simulink model "controllermodel"  (R2020b)
settings: Solver=FixedStepDiscrete  StartTime=0.0  StopTime=10.0  FixedStep=1/100  RelTol=1e-3
undefined symbols (not defined in the file or in its folder): DiscIntNeverNeededParam
libraries: simulink_extras x4, pid_lib x1
settings Model: Creator=janik  LastModifiedBy=Ralf Senger
settings OptimizationCC: DefaultParameterBehavior=Inlined  EnhancedBackFolding=on  PassReuseOutputArgsAs=Individual arguments  ZeroExternalMemoryAtStartup=off  ZeroInternalMemoryAtStartup=off  OptimizeBlockOrder=speed  DifferentSizesBufferReuse=on  OptimizationCustomize=off  EfficientTunableParamExpr=on
settings DebuggingCC: ParameterTunabilityLossMsg=error
settings SFSimCC: MATLABDynamicMemAlloc=off  SimTargetLang=C++
settings RTWCC: Description=Embedded Coder  SystemTargetFile=ert.tlc  GenCodeOnly=on  TemplateMakefile=ert_default_tmf  GenerateReport=on  Toolchain=GNU Tools for ARM Embedded Processors  LaunchReport=on  TargetLang=C++
settings CodeAppCC: ForceParamTrailComments=on  IgnoreCustomStorageClasses=off  OperatorAnnotations=on  SimulinkDataObjDesc=on  SFDataObjDesc=on  MATLABFcnDesc=on  InsertBlockDesc=on
settings ERTTargetCC: TargetLangStandard=C++03 (ISO)  GenerateSampleERTMain=on  CodeInterfacePackaging=C++ class  SupportVariableSizeSignals=on  InlinedParameterPlacement=NonHierarchical  RootIOFormat=Structure reference  ERTCustomFileTemplate=example_file_process.tlc

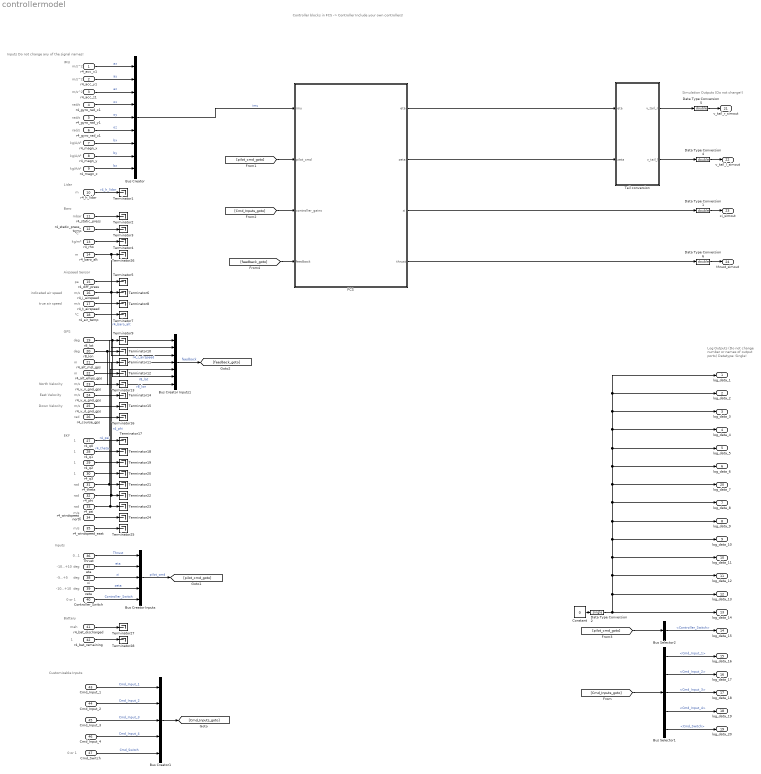
== system controllermodel ==
  note: EKF
  note: Lidar
  note: m/s
  note: Baro
  note: rad
  note: rad
  note: indicated air speed
  note: Inputs
      | Do not change any of the
      | signal names!
  note: m/s
  note: 1
  note: Controller blocks in FCS -> Controller
      |
      | Include your own controllers!
  note: -10...+10
  note: Log Outputs
      | (Do not change
      | number or names
      | of output ports)
      | Datatype: Single!
  note: deg
  note: pa
  note: East Velocity
  note: m
  note: kg/A/s²
  note: m
  note: m/s^2
  note: m/s^2
  note: true air speed
  note: Airpseed Sensor
  note: 1
  note: Inputs
  note: m/s
  note: mbar
  note: m
  note: deg
  note: kg/A/s²
  note: deg
  note: Battery
  note: rad/s
  note: 0 or 1
  note: 1
  note: rad/s
  note: mah
  note: Customizable Inputs
  note: m/s
  note: m/s
  note: m/s
  note: m/s^2
  note: North Velocity
  note: °C
  note: rad/s
  note: °C
  note: rad
  note: -5...+5
  note: m
  note: kg/A/s²
  note: 1
  note: 0...1
  note: deg
  note: rad
  note: Down Velocity
  note: IMU
  note: -10...+10
  note: deg
  note: 1
  note: Simulation Outputs
      | (Do not change!)
  note: 0 or 1
  note: GPS
  note: m/s
  note: kg/m³
  r4_acc_x1 : Inport  OutDataTypeStr=single  Unit=m/s^2  PortDimensions=1  SampleTime=1/50  Interpolate=off
  r4_acc_y1 : Inport  Port=2  OutDataTypeStr=single  Unit=m/s^2  PortDimensions=1  SampleTime=1/50  Interpolate=off
  r4_acc_z1 : Inport  Port=3  OutDataTypeStr=single  Unit=m/s^2  PortDimensions=1  SampleTime=1/50  Interpolate=off
  r4_gyro_rad_x1 : Inport  Port=4  OutDataTypeStr=single  Unit=rad/s  PortDimensions=1  SampleTime=1/50  Interpolate=off
  r4_gyro_rad_y1 : Inport  Port=5  OutDataTypeStr=single  Unit=rad/s  PortDimensions=1  SampleTime=1/50  Interpolate=off
  r4_gyro_rad_z1 : Inport  Port=6  OutDataTypeStr=single  Unit=rad/s  PortDimensions=1  SampleTime=1/50  Interpolate=off  LockScale=on
  r4_magn_x : Inport  Port=7  OutDataTypeStr=single  Unit=kg/A/s^2  PortDimensions=1  SampleTime=1/50  Interpolate=off
  r4_magn_y : Inport  Port=8  OutDataTypeStr=single  Unit=kg/A/s^2  PortDimensions=1  SampleTime=1/50  Interpolate=off
  r4_magn_z : Inport  Port=9  OutDataTypeStr=single  Unit=kg/A/s^2  PortDimensions=1  SampleTime=1/50  Interpolate=off
  r4_h_lidar : Inport  Port=10  OutDataTypeStr=single  Unit=m  PortDimensions=1  SampleTime=1/50  Interpolate=off
  r4_static_press : Inport  Port=11  OutDataTypeStr=single  Unit=mbar  PortDimensions=1  SampleTime=1/50  Interpolate=off
  r4_static_press_temp : Inport  Port=12  OutDataTypeStr=single  Unit=°C  PortDimensions=1  SampleTime=1/50  Interpolate=off
  r4_rho : Inport  Port=13  OutDataTypeStr=single  Unit=kg/m^3  PortDimensions=1  SampleTime=1/50  Interpolate=off
  r4_baro_alt : Inport  Port=14  OutDataTypeStr=single  Unit=m  PortDimensions=1  SampleTime=1/50  Interpolate=off
  r4_diff_press : Inport  Port=15  OutDataTypeStr=single  Unit=Pa  PortDimensions=1  SampleTime=1/50  Interpolate=off
  r4_i_airspeed : Inport  Port=16  OutDataTypeStr=single  Unit=m/s  PortDimensions=1  SampleTime=1/50  Interpolate=off
  r4_t_airspeed : Inport  Port=17  OutDataTypeStr=single  Unit=m/s  PortDimensions=1  SampleTime=1/50  Interpolate=off
  r4_air_temp : Inport  Port=18  OutDataTypeStr=single  Unit=°C  PortDimensions=1  SampleTime=1/50  Interpolate=off
  r8_lat : Inport  Port=19  OutDataTypeStr=double  Unit=deg  PortDimensions=1  SampleTime=1/50  Interpolate=off
  r8_lon : Inport  Port=20  OutDataTypeStr=double  Unit=deg  PortDimensions=1  SampleTime=1/50  Interpolate=off
  r4_alt_msl_gps : Inport  Port=21  OutDataTypeStr=single  Unit=m  PortDimensions=1  SampleTime=1/50  Interpolate=off
  r4_alt_ellips_gps : Inport  Port=22  OutDataTypeStr=single  Unit=m  PortDimensions=1  SampleTime=1/50  Interpolate=off
  r4_v_n_gnd_gps : Inport  Port=23  OutDataTypeStr=single  Unit=m/s  PortDimensions=1  SampleTime=1/50  Interpolate=off
  r4_v_e_gnd_gps : Inport  Port=24  OutDataTypeStr=single  Unit=m/s  PortDimensions=1  SampleTime=1/50  Interpolate=off
  r4_v_d_gnd_gps : Inport  Port=25  OutDataTypeStr=single  Unit=m/s  PortDimensions=1  SampleTime=1/50  Interpolate=off
  r4_course_gps : Inport  Port=26  OutDataTypeStr=single  Unit=rad  PortDimensions=1  SampleTime=1/50  Interpolate=off
  r4_q0 : Inport  Port=27  OutMin=[-1]  OutMax=[1]  OutDataTypeStr=single  Unit=1  PortDimensions=1  SampleTime=1/50  Interpolate=off
  r4_q1 : Inport  Port=28  OutMin=[-1]  OutMax=[1]  OutDataTypeStr=single  Unit=1  PortDimensions=1  SampleTime=1/50  Interpolate=off
  r4_q2 : Inport  Port=29  OutMin=[-1]  OutMax=[1]  OutDataTypeStr=single  Unit=1  PortDimensions=1  SampleTime=1/50  Interpolate=off
  r4_q3 : Inport  Port=30  OutMin=[-1]  OutMax=[1]  OutDataTypeStr=single  Unit=one  PortDimensions=1  SampleTime=1/50  Interpolate=off
  r4_theta : Inport  Port=31  OutDataTypeStr=single  Unit=rad  PortDimensions=1  SampleTime=1/50  Interpolate=off
  r4_phi : Inport  Port=32  OutDataTypeStr=single  Unit=rad  PortDimensions=1  SampleTime=1/50  Interpolate=off
  r4_psi : Inport  Port=33  OutDataTypeStr=single  Unit=rad  PortDimensions=1  SampleTime=1/50  Interpolate=off
  r4_windspeed_north : Inport  Port=34  OutDataTypeStr=single  Unit=m/s  PortDimensions=1  SampleTime=1/50  Interpolate=off
  r4_windspeed_east : Inport  Port=35  OutDataTypeStr=single  Unit=m/s  PortDimensions=1  SampleTime=1/50  Interpolate=off
  Thrust : Inport  Port=36  OutDataTypeStr=single  PortDimensions=1  SampleTime=1/50  Interpolate=off
  eta : Inport  Port=37  OutDataTypeStr=single  Unit=deg  PortDimensions=1  SampleTime=1/50  Interpolate=off
  xi : Inport  Port=38  OutDataTypeStr=single  Unit=deg  PortDimensions=1  SampleTime=1/50  Interpolate=off
  zeta : Inport  Port=39  OutDataTypeStr=single  Unit=deg  PortDimensions=1  SampleTime=1/50  Interpolate=off
  Controller_Switch : Inport  Port=40  OutDataTypeStr=single  PortDimensions=1  SampleTime=1/50  Interpolate=off
  r4_bat_discharged : Inport  Port=41  OutDataTypeStr=single  Unit=mA*hr  PortDimensions=1  SampleTime=1/50  Interpolate=off
  r4_bat_remaining : Inport  Port=42  OutDataTypeStr=single  PortDimensions=1  SampleTime=1/50  Interpolate=off
  Cmd_Input_1 : Inport  Port=43  OutDataTypeStr=single  PortDimensions=1  SampleTime=1/50  Interpolate=off
  Cmd_Input_2 : Inport  Port=44  OutDataTypeStr=single  PortDimensions=1  SampleTime=1/50  Interpolate=off
  Cmd_Input_3 : Inport  Port=45  OutDataTypeStr=single  PortDimensions=1  SampleTime=1/50  Interpolate=off
  Cmd_Input_4 : Inport  Port=46  OutDataTypeStr=single  PortDimensions=1  SampleTime=1/50  Interpolate=off
  Cmd_Switch : Inport  Port=47  OutDataTypeStr=single  PortDimensions=1  SampleTime=1/50  Interpolate=off
  Bus Creator : BusCreator  Inputs=9
  Bus Creator Inputs : BusCreator  Inputs=5
  Bus Creator Inputs1 : BusCreator  Inputs=7
  Bus Creator1 : BusCreator  Inputs=5
  Bus Selector1 : BusSelector  OutputSignals=Cmd_Input_1,Cmd_Input_2,Cmd_Input_3,Cmd_Input_4,Cmd_Switch
  Bus Selector2 : BusSelector  OutputSignals=Controller_Switch
  Constant : Constant  Value=0
  Data Type Conversion{1,4..6} (4 alike) : DataTypeConversion  OutDataTypeStr=double  RndMeth=Nearest
  Data Type Conversion2 : DataTypeConversion  OutDataTypeStr=single  RndMeth=Nearest
  FCS : Subsystem
  Tail conversion : Subsystem
  Terminator{1..28} (28 alike) : Terminator
  log_data_1 : Outport  OutDataTypeStr=single  VectorParamsAs1DForOutWhenUnconnected=off
  log_data_2 : Outport  Port=2  OutDataTypeStr=single  VectorParamsAs1DForOutWhenUnconnected=off
  log_data_3 : Outport  Port=3  OutDataTypeStr=single  VectorParamsAs1DForOutWhenUnconnected=off
  log_data_4 : Outport  Port=4  OutDataTypeStr=single  VectorParamsAs1DForOutWhenUnconnected=off
  log_data_5 : Outport  Port=5  OutDataTypeStr=single  VectorParamsAs1DForOutWhenUnconnected=off
  log_data_6 : Outport  Port=6  OutDataTypeStr=single  VectorParamsAs1DForOutWhenUnconnected=off
  log_data_8 : Outport  Port=7  OutDataTypeStr=single  VectorParamsAs1DForOutWhenUnconnected=off
  log_data_9 : Outport  Port=8  OutDataTypeStr=single  VectorParamsAs1DForOutWhenUnconnected=off
  log_data_10 : Outport  Port=9  OutDataTypeStr=single  VectorParamsAs1DForOutWhenUnconnected=off
  log_data_11 : Outport  Port=10  OutDataTypeStr=single  VectorParamsAs1DForOutWhenUnconnected=off
  log_data_12 : Outport  Port=11  OutDataTypeStr=single  VectorParamsAs1DForOutWhenUnconnected=off
  log_data_13 : Outport  Port=12  OutDataTypeStr=single  VectorParamsAs1DForOutWhenUnconnected=off
  log_data_14 : Outport  Port=13  OutDataTypeStr=single  VectorParamsAs1DForOutWhenUnconnected=off
  log_data_15 : Outport  Port=14  OutDataTypeStr=single  VectorParamsAs1DForOutWhenUnconnected=off
  log_data_16 : Outport  Port=15  OutDataTypeStr=single  VectorParamsAs1DForOutWhenUnconnected=off
  log_data_17 : Outport  Port=16  OutDataTypeStr=single  VectorParamsAs1DForOutWhenUnconnected=off
  log_data_18 : Outport  Port=17  OutDataTypeStr=single  VectorParamsAs1DForOutWhenUnconnected=off
  log_data_19 : Outport  Port=18  OutDataTypeStr=single  VectorParamsAs1DForOutWhenUnconnected=off
  log_data_20 : Outport  Port=19  OutDataTypeStr=single  VectorParamsAs1DForOutWhenUnconnected=off
  log_data_7 : Outport  Port=20  OutDataTypeStr=single  VectorParamsAs1DForOutWhenUnconnected=off
  v_tail_r_simout : Outport  Port=21  OutDataTypeStr=double  Unit=rad  VectorParamsAs1DForOutWhenUnconnected=off
  v_tail_l_simout : Outport  Port=22  OutDataTypeStr=double  Unit=rad  VectorParamsAs1DForOutWhenUnconnected=off
  xi_simout : Outport  Port=23  OutDataTypeStr=double  Unit=rad  VectorParamsAs1DForOutWhenUnconnected=off
  thrust_simout : Outport  Port=24  OutDataTypeStr=double  VectorParamsAs1DForOutWhenUnconnected=off
  wires:
  r4_bat_discharged/1 -> Terminator27/1
  [feedback_goto] -> FCS/4(feedback)
  Cmd_Switch/1 -> Bus Creator1/5  "Cmd_Switch"
  r4_theta/1 -> Bus Creator Inputs1/1, Terminator21/1  "r4_theta"
  Bus Selector1/5 -> log_data_20/1  "<Cmd_Switch>"
  r4_baro_alt/1 -> Bus Creator Inputs1/2, Terminator26/1  "r4_baro_alt"
  Data Type Conversion1/1 -> xi_simout/1
  r4_v_n_gnd_gps/1 -> Terminator13/1
  r4_static_press/1 -> Terminator2/1
  r4_h_lidar/1 -> Terminator1/1  "r4_h_lidar"
  Tail conversion/2(v_tail_l) -> Data Type Conversion4/1
  r4_q0/1 -> Terminator17/1
  FCS/4(thrust) -> Data Type Conversion6/1
  r4_alt_ellips_gps/1 -> Terminator12/1
  [Cmd_Inputs_goto] -> FCS/3(controller_gains)
  r4_gyro_rad_x1/1 -> Bus Creator/4  "ox"
  Data Type Conversion2/1 -> log_data_9/1, log_data_8/1, log_data_7/1, log_data_4/1, log_data_3/1, log_data_1/1, log_data_2/1, log_data_5/1, log_data_6/1, log_data_10/1, log_data_11/1, log_data_12/1, log_data_13/1, log_data_14/1
  r4_phi/1 -> Terminator22/1, Bus Creator Inputs1/4  "r4_phi"
  r4_i_airspeed/1 -> Bus Creator Inputs1/3, Terminator6/1  "r4_i_airspeed"
  FCS/2(zeta) -> Tail conversion/2(zeta)
  Bus Creator Inputs1/1 -> [feedback_goto]  "feedback"
  r4_psi/1 -> Terminator23/1, Bus Creator Inputs1/5  "r4_psi"
  r4_magn_x/1 -> Bus Creator/7  "bx"
  Data Type Conversion5/1 -> v_tail_r_simout/1
  r4_course_gps/1 -> Terminator16/1
  r4_magn_y/1 -> Bus Creator/8  "by"
  [pilot_cmd_goto] -> Bus Selector2/1
  r4_v_e_gnd_gps/1 -> Terminator14/1
  Bus Selector1/1 -> log_data_16/1  "<Cmd_Input_1>"
  Tail conversion/1(v_tail_r) -> Data Type Conversion5/1
  r4_t_airspeed/1 -> Terminator8/1
  r4_acc_y1/1 -> Bus Creator/2  "ay"
  Cmd_Input_1/1 -> Bus Creator1/1  "Cmd_Input_1"
  FCS/1(eta) -> Tail conversion/1(eta)
  Bus Selector1/4 -> log_data_19/1  "<Cmd_Input_4>"
  xi/1 -> Bus Creator Inputs/3  "xi"
  r4_windspeed_north/1 -> Terminator24/1
  r4_gyro_rad_z1/1 -> Bus Creator/6  "oz"
  eta/1 -> Bus Creator Inputs/2  "eta"
  Bus Selector2/1 -> log_data_15/1  "<Controller_Switch>"
  zeta/1 -> Bus Creator Inputs/4  "zeta"
  Bus Creator Inputs/1 -> [pilot_cmd_goto]  "pilot_cmd"
  Cmd_Input_2/1 -> Bus Creator1/2  "Cmd_Input_2"
  Data Type Conversion4/1 -> v_tail_l_simout/1
  r8_lat/1 -> Terminator9/1, Bus Creator Inputs1/6  "r8_lat"
  Cmd_Input_3/1 -> Bus Creator1/3  "Cmd_Input_3"
  r4_q1/1 -> Terminator18/1
  r4_q3/1 -> Terminator20/1
  r4_rho/1 -> Terminator4/1
  Data Type Conversion6/1 -> thrust_simout/1
  Controller_Switch/1 -> Bus Creator Inputs/5  "Controller_Switch"
  [pilot_cmd_goto] -> FCS/2(pilot_cmd)
  Thrust/1 -> Bus Creator Inputs/1  "Thrust"
  Cmd_Input_4/1 -> Bus Creator1/4  "Cmd_Input_4"
  FCS/3(xi) -> Data Type Conversion1/1
  r4_air_temp/1 -> Terminator7/1
  r4_acc_z1/1 -> Bus Creator/3  "az"
  r4_acc_x1/1 -> Bus Creator/1  "ax"
  r4_static_press_temp/1 -> Terminator3/1
  r8_lon/1 -> Terminator10/1, Bus Creator Inputs1/7  "r8_lon"
  Constant/1 -> Data Type Conversion2/1
  Bus Creator/1 -> FCS/1(imu)  "imu"
  r4_windspeed_east/1 -> Terminator25/1
  r4_bat_remaining/1 -> Terminator28/1
  Bus Selector1/2 -> log_data_17/1  "<Cmd_Input_2>"
  r4_magn_z/1 -> Bus Creator/9  "bz"
  r4_q2/1 -> Terminator19/1
  [Cmd_Inputs_goto] -> Bus Selector1/1
  r4_gyro_rad_y1/1 -> Bus Creator/5  "oy"
  r4_diff_press/1 -> Terminator5/1
  Bus Selector1/3 -> log_data_18/1  "<Cmd_Input_3>"
  r4_alt_msl_gps/1 -> Terminator11/1
  r4_v_d_gnd_gps/1 -> Terminator15/1
  Bus Creator1/1 -> [Cmd_Inputs_goto]

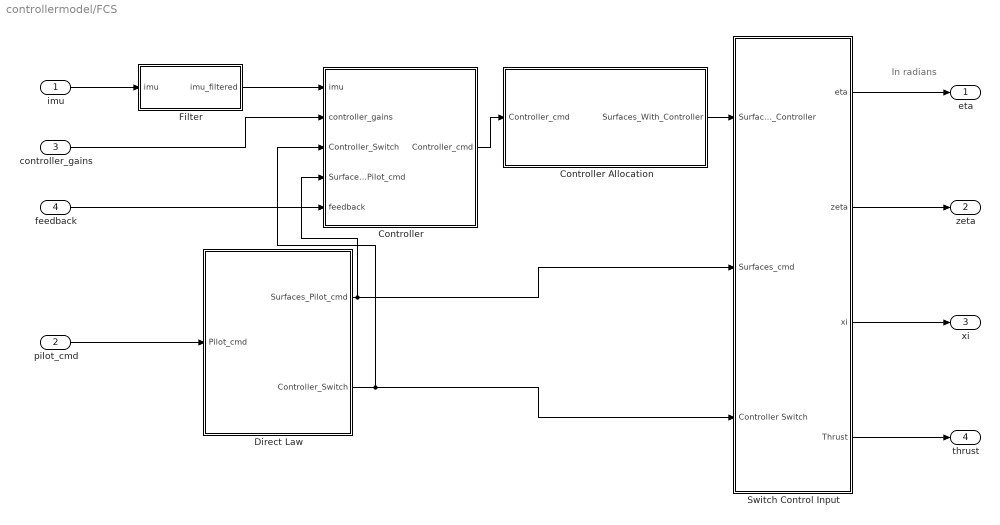
== system controllermodel/FCS ==
  note: In radians
  imu : Inport
  pilot_cmd : Inport  Port=2
  controller_gains : Inport  Port=3
  feedback : Inport  Port=4
  Controller : Subsystem
  Controller Allocation : Subsystem
  Direct Law : Subsystem
  Filter : Subsystem
  Switch Control Input : Subsystem
  eta : Outport  Unit=rad
  zeta : Outport  Port=2  Unit=rad
  xi : Outport  Port=3  Unit=rad
  thrust : Outport  Port=4  Unit=rad
  wires:
  Controller Allocation/1(Surfaces_With_Controller) -> Switch Control Input/1(Surfaces_With_Controller)
  pilot_cmd/1 -> Direct Law/1(Pilot_cmd)
  imu/1 -> Filter/1(imu)
  Switch Control Input/4(Thrust) -> thrust/1
  Switch Control Input/2(zeta) -> zeta/1
  Switch Control Input/1(eta) -> eta/1
  Switch Control Input/3(xi) -> xi/1
  Filter/1(imu_filtered) -> Controller/1(imu)
  Direct Law/2(Controller_Switch) -> Switch Control Input/3(Controller Switch), Controller/3(Controller_Switch)
  controller_gains/1 -> Controller/2(controller_gains)
  Direct Law/1(Surfaces_Pilot_cmd) -> Switch Control Input/2(Surfaces_cmd), Controller/4(Surfaces_Pilot_cmd)
  Controller/1(Controller_cmd) -> Controller Allocation/1(Controller_cmd)
  feedback/1 -> Controller/5(feedback)

== system controllermodel/Tail conversion ==
  eta : Inport  Unit=rad
  zeta : Inport  Port=2  Unit=rad
  Add1 : Sum  OutDataTypeStr=double
  Add2 : Sum  Inputs=+-  InputSameDT=on  OutDataTypeStr=double
  v_tail_r : Outport  Unit=rad
  v_tail_l : Outport  Port=2  Unit=rad
  wires:
  Add1/1 -> v_tail_l/1
  Add2/1 -> v_tail_r/1
  zeta/1 -> Add2/2, Add1/2
  eta/1 -> Add2/1, Add1/1

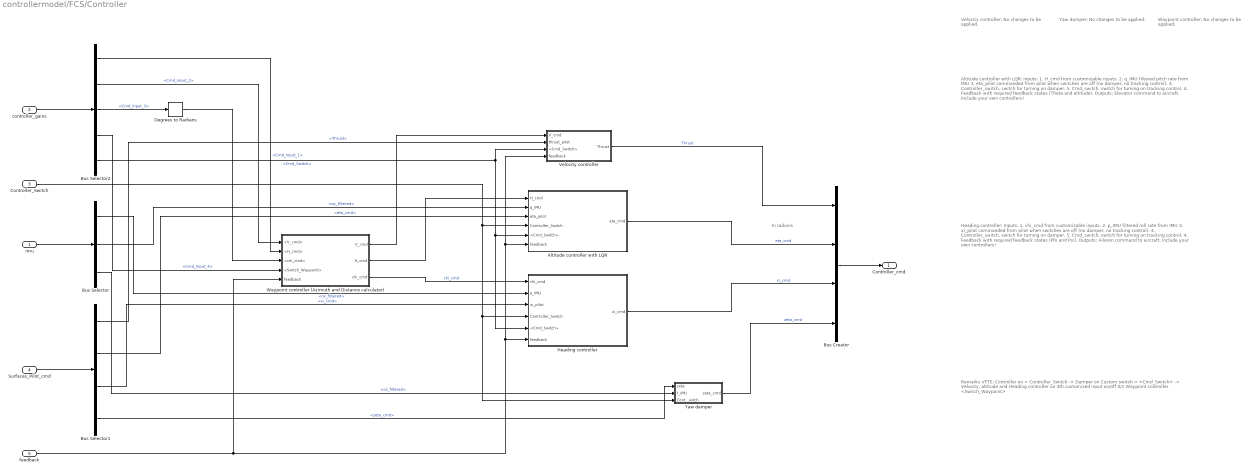
== system controllermodel/FCS/Controller ==
  note: Remarks VFTE:
      |
      | Controller on = Controller_Switch -> Damper on
      | Custom switch = <Cmd_Switch> -> Velocity, altitude and Heading controller on
      | 4th customized input on/off 0/1 Waypoint controller <Switch_Waypoint>
  note: In radians
  note: Veloctiy controller:
      |
      | No changes to be applied.
  note: Altitude controller with LQR:
      |
      | Inputs:
      |
      | 1. H_cmd from customizable inputs.
      | 2. q_IMU filtered pitch rate from IMU
      | 3. eta_pilot commanded from pilot when switches are off (no damper, no tracking control).
      | 4. Controller_switch, switch for turning on damper.
      | 5. Cmd_switch, switch for turning on tracking control.
      | 4. Feedback with required feedback states (Theta and altitude).
      |
      | Outputs:
      |
      | Elevator command to aircraft.
      |
      | Include your own controllers!
  note: Heading controller:
      |
      | Inputs:
      |
      | 1. chi_cmd from customizable inputs.
      | 2. p_IMU filtered roll rate from IMU
      | 3. xi_pilot commanded from pilot when switches are off (no damper, no tracking control).
      | 4. Controller_switch, switch for turning on damper.
      | 5. Cmd_switch, switch for turning on tracking control.
      | 4. Feedback with required feedback states (Phi and Psi).
      |
      | Outputs:
      |
      | Aileron command to aircraft.
      |
      | Include your own controllers!
  note: Yaw damper:
      |
      | No changes to be applied.
  note: Waypoint controller:
      |
      | No changes to be applied.
  imu : Inport
  controller_gains : Inport  Port=2
  Controller_Switch : Inport  Port=3
  Surfaces_Pilot_cmd : Inport  Port=4
  feedback : Inport  Port=5
  Altitude controller with LQR : Subsystem
  Bus Creator : BusCreator  Inputs=4
  Bus Selector : BusSelector  OutputSignals=ox_filtered,oy_filtered,oz_filtered
  Bus Selector1 : BusSelector  OutputSignals=Thrust,eta_cmd,xi_cmd,zeta_cmd
  Bus Selector2 : BusSelector  OutputSignals=Cmd_Input_1,Cmd_Input_2,Cmd_Input_3,Cmd_Input_4,Cmd_Switch
  Degrees to Radians : simulink_extras/Transformations/Degrees to Radians
  Heading controller : Subsystem
  Velocity controller : Subsystem
  Waypoint controller (Azimuth and Distance calculator) : Subsystem
  Yaw damper : Subsystem
  Controller_cmd : Outport
  wires:
  Bus Creator/1 -> Controller_cmd/1
  controller_gains/1 -> Bus Selector2/1
  Altitude controller with LQR/1(eta_cmd) -> Bus Creator/2  "eta_cmd"
  Bus Selector/3 -> Yaw damper/2(r_IMU)  "<oz_filtered>"
  Bus Selector/1 -> Heading controller/2(p_IMU)  "<ox_filtered>"
  Bus Selector/2 -> Altitude controller with LQR/2(q_IMU)  "<oy_filtered>"
  imu/1 -> Bus Selector/1
  Controller_Switch/1 -> Altitude controller with LQR/4(Controller_Switch), Yaw damper/3(Controller_Switch), Heading controller/4(Controller_Switch)
  Surfaces_Pilot_cmd/1 -> Bus Selector1/1
  Bus Selector1/2 -> Altitude controller with LQR/3(eta_pilot)  "<eta_cmd>"
  Bus Selector1/1 -> Velocity controller/2(thrust_pilot)  "<Thrust>"
  Bus Selector1/3 -> Heading controller/3(xi_pilot)  "<xi_cmd>"
  Bus Selector1/4 -> Yaw damper/1(zeta)  "<zeta_cmd>"
  feedback/1 -> Waypoint controller (Azimuth and Distance calculator)/5(feedback), Velocity controller/4(feedback), Altitude controller with LQR/6(feedback), Heading controller/6(feedback)
  Bus Selector2/1 -> Waypoint controller (Azimuth and Distance calculator)/2(<H_cmd>)  "<Cmd_Input_1>"
  Bus Selector2/2 -> Waypoint controller (Azimuth and Distance calculator)/1(<V_cmd>)  "<Cmd_Input_2>"
  Bus Selector2/3 -> Degrees to Radians/1  "<Cmd_Input_3>"
  Bus Selector2/4 -> Waypoint controller (Azimuth and Distance calculator)/4(<Switch_Waypoint>)  "<Cmd_Input_4>"
  Bus Selector2/5 -> Heading controller/5(<Cmd_Switch>), Altitude controller with LQR/5(<Cmd_Switch>), Velocity controller/3(<Cmd_Switch>)  "<Cmd_Switch>"
  Velocity controller/1(Thrust) -> Bus Creator/1  "Thrust"
  Heading controller/1(xi_cmd) -> Bus Creator/3  "xi_cmd"
  Yaw damper/1(zeta_cmd) -> Bus Creator/4  "zeta_cmd"
  Degrees to Radians/1 -> Waypoint controller (Azimuth and Distance calculator)/3(<chi_cmd>)
  Waypoint controller (Azimuth and Distance calculator)/3(chi_cmd) -> Heading controller/1(chi_cmd)  "chi_cmd"
  Waypoint controller (Azimuth and Distance calculator)/1(V_cmd) -> Velocity controller/1(V_cmd)
  Waypoint controller (Azimuth and Distance calculator)/2(H_cmd) -> Altitude controller with LQR/1(H_cmd)

== system controllermodel/FCS/Controller Allocation ==
  note: Do not change signal names
      | or saturation
  Controller_cmd : Inport
  Bus Creator : BusCreator  Inputs=4
  Bus Selector1 : BusSelector  OutputSignals=Thrust,eta_cmd,xi_cmd,zeta_cmd
  Saturation : Saturate  UpperLimit=deg2rad(10)  LowerLimit=deg2rad(-20)
  Saturation1 : Saturate  UpperLimit=deg2rad(5)  LowerLimit=deg2rad(-5)
  Saturation2 : Saturate  UpperLimit=deg2rad(10)  LowerLimit=deg2rad(-10)
  Saturation3 : Saturate  UpperLimit=1  LowerLimit=0
  Surfaces_With_Controller : Outport
  wires:
  Bus Creator/1 -> Surfaces_With_Controller/1
  Controller_cmd/1 -> Bus Selector1/1
  Bus Selector1/4 -> Saturation2/1  "<zeta_cmd>"
  Bus Selector1/3 -> Saturation1/1  "<xi_cmd>"
  Bus Selector1/2 -> Saturation/1  "<eta_cmd>"
  Bus Selector1/1 -> Saturation3/1  "<Thrust>"
  Saturation/1 -> Bus Creator/2  "eta_cmd"
  Saturation1/1 -> Bus Creator/3  "xi_cmd"
  Saturation2/1 -> Bus Creator/4  "zeta_cmd"
  Saturation3/1 -> Bus Creator/1  "Thrust"

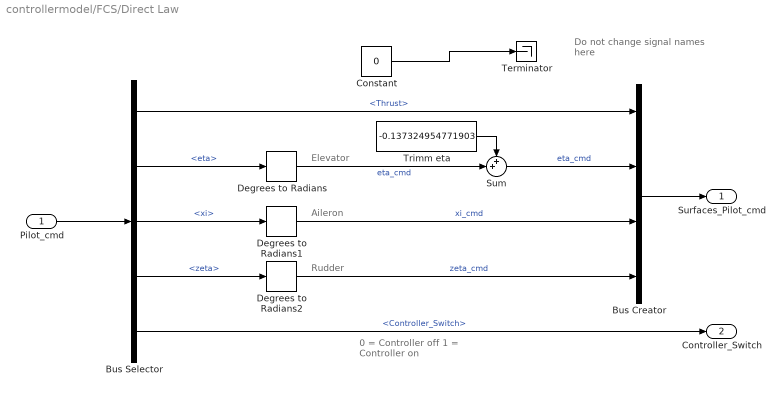
== system controllermodel/FCS/Direct Law ==
  note: Elevator
  note: 0 = Controller off
      | 1 = Controller on
  note: Do not change
      | signal names
      | here
  note: Aileron
  note: Rudder
  Pilot_cmd : Inport
  Bus Creator : BusCreator  Inputs=4
  Bus Selector : BusSelector  OutputSignals=Thrust,eta,xi,zeta,Controller_Switch
  Constant : Constant  Value=0
  Degrees to Radians : simulink_extras/Transformations/Degrees to Radians
  Degrees to Radians1 : simulink_extras/Transformations/Degrees to Radians
  Degrees to Radians2 : simulink_extras/Transformations/Degrees to Radians
  Sum : Sum  Inputs=++|
  Terminator : Terminator
  Trimm eta : Constant  Description=trim thrust  Value=-0.137324954771903  OutDataTypeStr=double
  Surfaces_Pilot_cmd : Outport
  Controller_Switch : Outport  Port=2
  wires:
  Pilot_cmd/1 -> Bus Selector/1
  Bus Selector/1 -> Bus Creator/1  "<Thrust>"
  Bus Selector/2 -> Degrees to Radians/1  "<eta>"
  Bus Selector/4 -> Degrees to Radians2/1  "<zeta>"
  Bus Selector/3 -> Degrees to Radians1/1  "<xi>"
  Bus Selector/5 -> Controller_Switch/1  "<Controller_Switch>"
  Bus Creator/1 -> Surfaces_Pilot_cmd/1
  Sum/1 -> Bus Creator/2  "eta_cmd"
  Degrees to Radians1/1 -> Bus Creator/3  "xi_cmd"
  Degrees to Radians2/1 -> Bus Creator/4  "zeta_cmd"
  Degrees to Radians/1 -> Sum/2  "eta_cmd"
  Trimm eta/1 -> Sum/1
  Constant/1 -> Terminator/1

== system controllermodel/FCS/Filter ==
  imu : Inport
  Bus Creator : BusCreator  Inputs=3
  Bus Selector : BusSelector  OutputSignals=ox,oy,oz
  ox_Filter : Subsystem
  oy_Filter : Subsystem
  oz_Filter : Subsystem
  imu_filtered : Outport
  wires:
  imu/1 -> Bus Selector/1
  Bus Selector/1 -> ox_Filter/1(<ox>)  "<ox>"
  ox_Filter/1(ox_filtered) -> Bus Creator/1  "ox_filtered"
  Bus Selector/2 -> oy_Filter/1(<oy>)  "<oy>"
  oy_Filter/1(oy_filtered) -> Bus Creator/2  "oy_filtered"
  Bus Selector/3 -> oz_Filter/1(<oz>)  "<oz>"
  oz_Filter/1(oz_filtered) -> Bus Creator/3  "oz_filtered"
  Bus Creator/1 -> imu_filtered/1

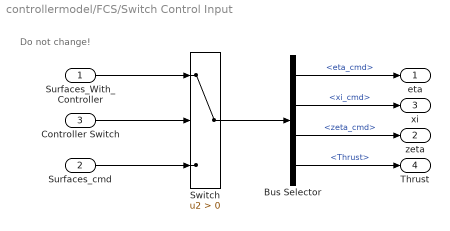
== system controllermodel/FCS/Switch Control Input ==
  note: Do not change!
  Surfaces_With_Controller : Inport
  Surfaces_cmd : Inport  Port=2
  Controller Switch : Inport  Port=3
  Bus Selector : BusSelector  OutputSignals=eta_cmd,xi_cmd,zeta_cmd,Thrust
  Switch : Switch  Criteria=u2 > Threshold
  eta : Outport
  zeta : Outport  Port=2
  xi : Outport  Port=3
  Thrust : Outport  Port=4
  wires:
  Surfaces_With_Controller/1 -> Switch/1
  Controller Switch/1 -> Switch/2
  Surfaces_cmd/1 -> Switch/3
  Switch/1 -> Bus Selector/1
  Bus Selector/1 -> eta/1  "<eta_cmd>"
  Bus Selector/2 -> xi/1  "<xi_cmd>"
  Bus Selector/3 -> zeta/1  "<zeta_cmd>"
  Bus Selector/4 -> Thrust/1  "<Thrust>"

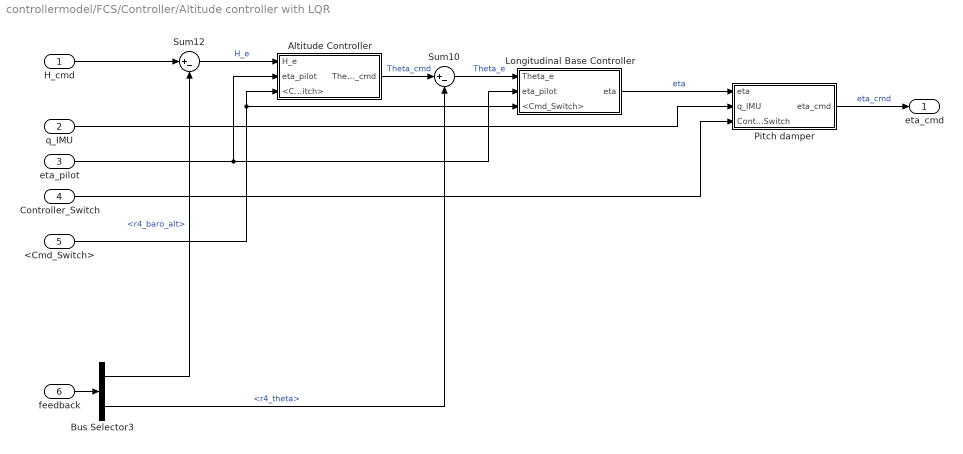
== system controllermodel/FCS/Controller/Altitude controller with LQR ==
  H_cmd : Inport
  q_IMU : Inport  Port=2
  eta_pilot : Inport  Port=3
  Controller_Switch : Inport  Port=4
  <Cmd_Switch> : Inport  Port=5
  feedback : Inport  Port=6
  Altitude Controller : Subsystem
  Bus Selector3 : BusSelector  OutputSignals=r4_baro_alt,r4_theta
  Longitudinal Base Controller : Subsystem
  Pitch damper : Subsystem
  Sum10 : Sum  Inputs=|+-
  Sum12 : Sum  Inputs=|+-
  eta_cmd : Outport
  wires:
  H_cmd/1 -> Sum12/1
  Pitch damper/1(eta_cmd) -> eta_cmd/1  "eta_cmd"
  Longitudinal Base Controller/1(eta) -> Pitch damper/1(eta)  "eta"
  Altitude Controller/1(Theta_cmd) -> Sum10/1  "Theta_cmd"
  Sum10/1 -> Longitudinal Base Controller/1(Theta_e)  "Theta_e"
  Sum12/1 -> Altitude Controller/1(H_e)  "H_e"
  q_IMU/1 -> Pitch damper/2(q_IMU)
  eta_pilot/1 -> Altitude Controller/2(eta_pilot), Longitudinal Base Controller/2(eta_pilot)
  Controller_Switch/1 -> Pitch damper/3(Controller_Switch)
  <Cmd_Switch>/1 -> Longitudinal Base Controller/3(<Cmd_Switch>), Altitude Controller/3(<Cmd_Switch>)
  feedback/1 -> Bus Selector3/1
  Bus Selector3/2 -> Sum10/2  "<r4_theta>"
  Bus Selector3/1 -> Sum12/2  "<r4_baro_alt>"

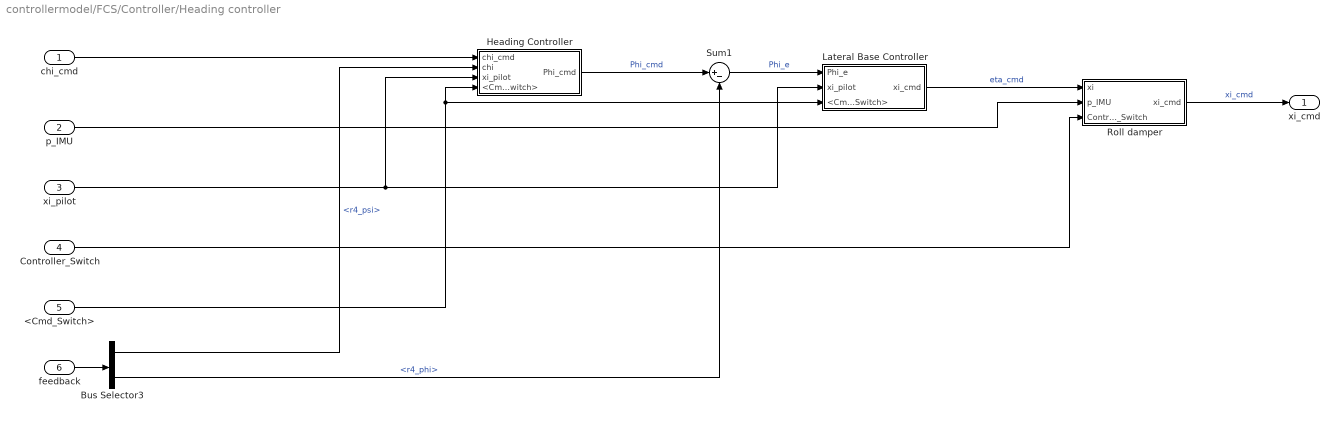
== system controllermodel/FCS/Controller/Heading controller ==
  chi_cmd : Inport
  p_IMU : Inport  Port=2
  xi_pilot : Inport  Port=3
  Controller_Switch : Inport  Port=4
  <Cmd_Switch> : Inport  Port=5
  feedback : Inport  Port=6
  Bus Selector3 : BusSelector  OutputSignals=r4_psi,r4_phi
  Heading Controller : Subsystem
  Lateral Base Controller : Subsystem
  Roll damper : Subsystem
  Sum1 : Sum  Inputs=|+-
  xi_cmd : Outport
  wires:
  Heading Controller/1(Phi_cmd) -> Sum1/1  "Phi_cmd"
  Roll damper/1(xi_cmd) -> xi_cmd/1  "xi_cmd"
  Lateral Base Controller/1(xi_cmd) -> Roll damper/1(xi)  "eta_cmd"
  Sum1/1 -> Lateral Base Controller/1(Phi_e)  "Phi_e"
  chi_cmd/1 -> Heading Controller/1(chi_cmd)
  p_IMU/1 -> Roll damper/2(p_IMU)
  xi_pilot/1 -> Heading Controller/3(xi_pilot), Lateral Base Controller/2(xi_pilot)
  Controller_Switch/1 -> Roll damper/3(Controller_Switch)
  <Cmd_Switch>/1 -> Heading Controller/4(<Cmd_Switch>), Lateral Base Controller/3(<Cmd_Switch>)
  Bus Selector3/2 -> Sum1/2  "<r4_phi>"
  feedback/1 -> Bus Selector3/1
  Bus Selector3/1 -> Heading Controller/2(chi)  "<r4_psi>"

== system controllermodel/FCS/Controller/Velocity controller ==
  V_cmd : Inport
  thrust_pilot : Inport  Port=2
  <Cmd_Switch> : Inport  Port=3
  feedback : Inport  Port=4
  Bus Selector3 : BusSelector  OutputSignals=r4_i_airspeed
  Sum14 : Sum  Inputs=|+-
  Velocity controller : Subsystem
  Thrust : Outport
  wires:
  Sum14/1 -> Velocity controller/1(V_e)  "V_e"
  Velocity controller/1(Thrust) -> Thrust/1  "Thrust"
  V_cmd/1 -> Sum14/1
  thrust_pilot/1 -> Velocity controller/2(thrust_pilot)
  <Cmd_Switch>/1 -> Velocity controller/3(<Cmd_Switch>)
  Bus Selector3/1 -> Sum14/2  "<r4_i_airspeed>"
  feedback/1 -> Bus Selector3/1

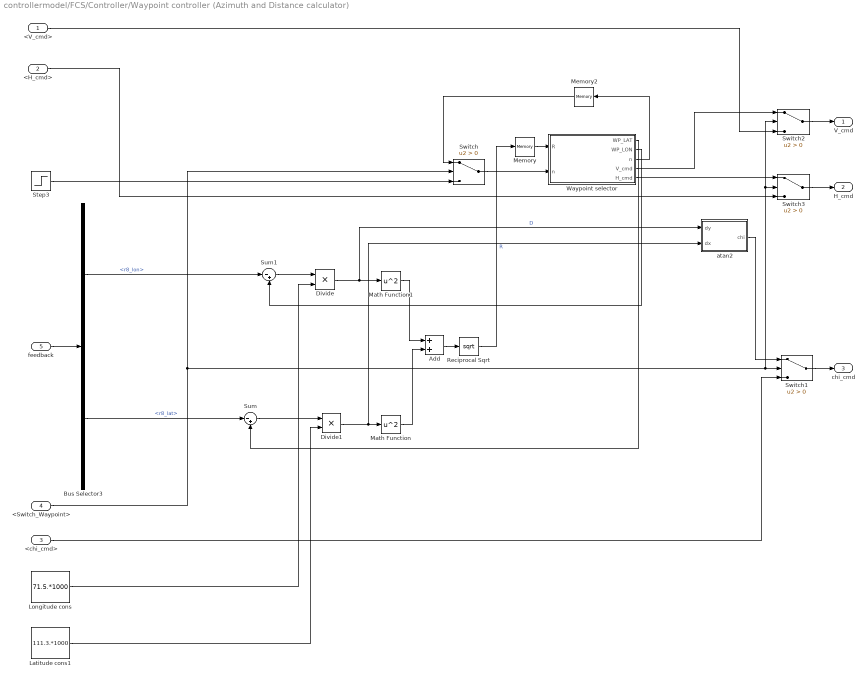
== system controllermodel/FCS/Controller/Waypoint controller (Azimuth and Distance calculator) ==
  <V_cmd> : Inport
  <H_cmd> : Inport  Port=2
  <chi_cmd> : Inport  Port=3
  <Switch_Waypoint> : Inport  Port=4
  feedback : Inport  Port=5
  Add : Sum
  Bus Selector3 : BusSelector  OutputSignals=r8_lon,r8_lat
  Divide : Product
  Divide1 : Product
  Latitude cons1 : Constant  Value=111.3.*1000
  Longitude cons : Constant  Value=71.5.*1000
  Math Function : Math  Operator=square  SaturateOnIntegerOverflow=on
  Math Function1 : Math  Operator=square  SaturateOnIntegerOverflow=on
  Memory : Memory
  Memory2 : Memory
  Reciprocal Sqrt : Sqrt  SaturateOnIntegerOverflow=on
  Step3 : Step  Time=0  Before=1  SampleTime=0.01
  Sum : Sum  Inputs=|-+
  Sum1 : Sum  Inputs=|-+
  Switch{,1..3} (4 alike) : Switch  Criteria=u2 > Threshold
  Waypoint selector : MATLAB Function  TreatAsAtomicUnit=on
  atan2 : MATLAB Function  TreatAsAtomicUnit=on
  V_cmd : Outport
  H_cmd : Outport  Port=2
  chi_cmd : Outport  Port=3
  wires:
  Longitude cons/1 -> Divide/2
  Sum1/1 -> Divide/1
  Sum/1 -> Divide1/1
  Latitude cons1/1 -> Divide1/2
  Divide1/1 -> atan2/2(dx), Math Function/1
  Divide/1 -> atan2/1(dy), Math Function1/1  "D"
  Math Function/1 -> Add/2
  Math Function1/1 -> Add/1
  Add/1 -> Reciprocal Sqrt/1
  Reciprocal Sqrt/1 -> Memory/1  "R"
  Waypoint selector/2(WP_LON) -> Sum1/2
  Switch/1 -> Waypoint selector/2("n ")
  Memory/1 -> Waypoint selector/1(R)
  Waypoint selector/1(WP_LAT) -> Sum/2
  Waypoint selector/3(n) -> Memory2/1
  Memory2/1 -> Switch/1
  Step3/1 -> Switch/3
  atan2/1(chi) -> Switch1/1
  Switch1/1 -> chi_cmd/1
  <Switch_Waypoint>/1 -> Switch2/2, Switch3/2, Switch1/2, Switch/2
  <chi_cmd>/1 -> Switch1/3
  Bus Selector3/1 -> Sum1/1  "<r8_lon>"
  Bus Selector3/2 -> Sum/1  "<r8_lat>"
  feedback/1 -> Bus Selector3/1
  Switch2/1 -> V_cmd/1
  Switch3/1 -> H_cmd/1
  <V_cmd>/1 -> Switch2/3
  <H_cmd>/1 -> Switch3/3
  Waypoint selector/4(V_cmd) -> Switch2/1
  Waypoint selector/5(H_cmd) -> Switch3/1

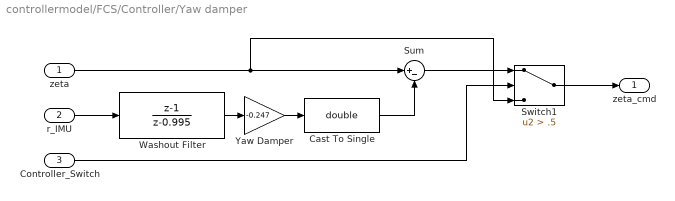
== system controllermodel/FCS/Controller/Yaw damper ==
  zeta : Inport
  r_IMU : Inport  Port=2
  Controller_Switch : Inport  Port=3
  Cast To Single : DataTypeConversion  OutDataTypeStr=double
  Sum : Sum  Inputs=|+-
  Switch1 : Switch  Criteria=u2 > Threshold  Threshold=.5
  Washout Filter : DiscreteTransferFcn  Numerator=[1 -1]  Denominator=[1 -0.995]  OutDataTypeStr=Inherit: Same as input
  Yaw Damper : Gain  Gain=-0.247  OutDataTypeStr=Inherit: Same as input
  zeta_cmd : Outport
  wires:
  r_IMU/1 -> Washout Filter/1
  Sum/1 -> Switch1/1
  zeta/1 -> Switch1/3, Sum/1
  Switch1/1 -> zeta_cmd/1
  Controller_Switch/1 -> Switch1/2
  Yaw Damper/1 -> Cast To Single/1
  Washout Filter/1 -> Yaw Damper/1
  Cast To Single/1 -> Sum/2

== system controllermodel/FCS/Filter/ox_Filter ==
  <ox> : Inport
  Discrete-Time Integrator : DiscreteIntegrator  SampleTime=-1  ICPrevOutput=DiscIntNeverNeededParam  ICPrevScaledInput=DiscIntNeverNeededParam
  Filter_A : Gain  Gain=-0.3183
  Filter_B : Gain  Gain=0.5
  Filter_C : Gain  Gain=0.6366
  Sum : Sum  Inputs=|++
  ox_filtered : Outport
  wires:
  <ox>/1 -> Filter_B/1
  Filter_C/1 -> ox_filtered/1
  Filter_B/1 -> Sum/1
  Discrete-Time Integrator/1 -> Filter_A/1, Filter_C/1
  Filter_A/1 -> Sum/2
  Sum/1 -> Discrete-Time Integrator/1

== system controllermodel/FCS/Filter/oy_Filter ==
  <oy> : Inport
  Discrete-Time Integrator : DiscreteIntegrator  SampleTime=-1  ICPrevOutput=DiscIntNeverNeededParam  ICPrevScaledInput=DiscIntNeverNeededParam
  Filter_A : Gain  Gain=-0.3183
  Filter_B : Gain  Gain=0.5
  Filter_C : Gain  Gain=0.6366
  Sum : Sum  Inputs=|++
  oy_filtered : Outport
  wires:
  <oy>/1 -> Filter_B/1
  Filter_C/1 -> oy_filtered/1
  Filter_B/1 -> Sum/1
  Discrete-Time Integrator/1 -> Filter_A/1, Filter_C/1
  Filter_A/1 -> Sum/2
  Sum/1 -> Discrete-Time Integrator/1

== system controllermodel/FCS/Filter/oz_Filter ==
  <oz> : Inport
  Discrete-Time Integrator : DiscreteIntegrator  SampleTime=-1  ICPrevOutput=DiscIntNeverNeededParam  ICPrevScaledInput=DiscIntNeverNeededParam
  Filter_A : Gain  Gain=-0.3183
  Filter_B : Gain  Gain=0.5
  Filter_C : Gain  Gain=0.6366
  Sum : Sum  Inputs=|++
  oz_filtered : Outport
  wires:
  Sum/1 -> Discrete-Time Integrator/1
  Filter_A/1 -> Sum/2
  Discrete-Time Integrator/1 -> Filter_C/1, Filter_A/1
  Filter_B/1 -> Sum/1
  Filter_C/1 -> oz_filtered/1
  <oz>/1 -> Filter_B/1

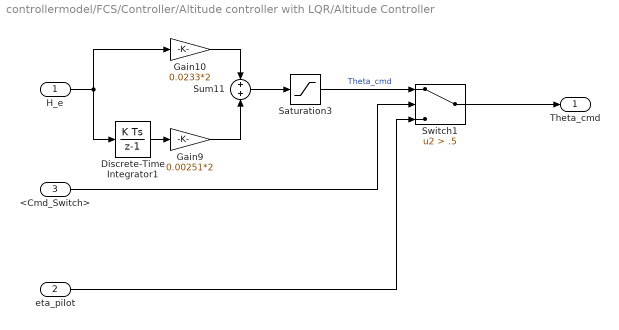
== system controllermodel/FCS/Controller/Altitude controller with LQR/Altitude Controller ==
  H_e : Inport
  eta_pilot : Inport  Port=2
  <Cmd_Switch> : Inport  Port=3
  Discrete-Time Integrator1 : DiscreteIntegrator  InitialCondition=0.029323438079024/(0.00251*2)  SampleTime=0.01  LimitOutput=on  UpperSaturationLimit=20  LowerSaturationLimit=-20  ICPrevOutput=DiscIntNeverNeededParam  ICPrevScaledInput=DiscIntNeverNeededParam
  Gain10 : Gain  Gain=0.0233*2
  Gain9 : Gain  Gain=0.00251*2
  Saturation3 : Saturate  UpperLimit=30*(pi/180)  LowerLimit=-30*(pi/180)
  Sum11 : Sum
  Switch1 : Switch  Criteria=u2 > Threshold  Threshold=.5
  Theta_cmd : Outport
  wires:
  H_e/1 -> Discrete-Time Integrator1/1, Gain10/1
  Gain10/1 -> Sum11/1
  Discrete-Time Integrator1/1 -> Gain9/1
  Sum11/1 -> Saturation3/1
  Saturation3/1 -> Switch1/1  "Theta_cmd"
  Gain9/1 -> Sum11/2
  Switch1/1 -> Theta_cmd/1
  <Cmd_Switch>/1 -> Switch1/2
  eta_pilot/1 -> Switch1/3

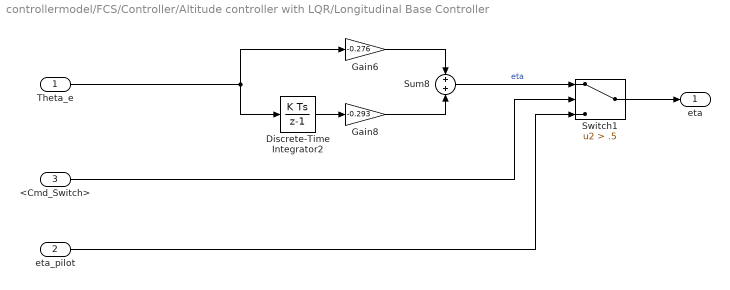
== system controllermodel/FCS/Controller/Altitude controller with LQR/Longitudinal Base Controller ==
  Theta_e : Inport
  eta_pilot : Inport  Port=2
  <Cmd_Switch> : Inport  Port=3
  Discrete-Time Integrator2 : DiscreteIntegrator  InitialCondition=-0.137324954771903/-0.293  SampleTime=0.01  LimitOutput=on  UpperSaturationLimit=30*(pi/180)  LowerSaturationLimit=-30*(pi/180)  ICPrevOutput=DiscIntNeverNeededParam  ICPrevScaledInput=DiscIntNeverNeededParam
  Gain6 : Gain  Gain=-0.276
  Gain8 : Gain  Gain=-0.293
  Sum8 : Sum
  Switch1 : Switch  Criteria=u2 > Threshold  Threshold=.5
  eta : Outport
  wires:
  Discrete-Time Integrator2/1 -> Gain8/1
  Gain8/1 -> Sum8/2
  Theta_e/1 -> Discrete-Time Integrator2/1, Gain6/1
  Gain6/1 -> Sum8/1
  Sum8/1 -> Switch1/1  "eta"
  <Cmd_Switch>/1 -> Switch1/2
  Switch1/1 -> eta/1
  eta_pilot/1 -> Switch1/3

== system controllermodel/FCS/Controller/Altitude controller with LQR/Pitch damper ==
  eta : Inport
  q_IMU : Inport  Port=2
  Controller_Switch : Inport  Port=3
  Gain : Gain  Gain=-0.125
  Sum : Sum  Inputs=|+-
  Switch1 : Switch  Criteria=u2 > Threshold  Threshold=.5
  eta_cmd : Outport
  wires:
  q_IMU/1 -> Gain/1
  Gain/1 -> Sum/2
  Sum/1 -> Switch1/1
  eta/1 -> Switch1/3, Sum/1
  Switch1/1 -> eta_cmd/1
  Controller_Switch/1 -> Switch1/2

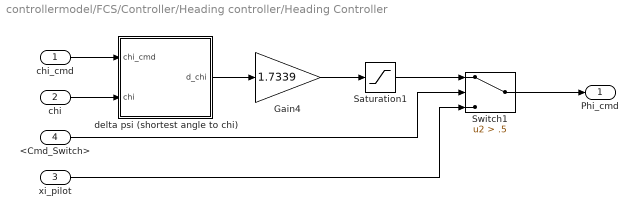
== system controllermodel/FCS/Controller/Heading controller/Heading Controller ==
  chi_cmd : Inport
  chi : Inport  Port=2
  xi_pilot : Inport  Port=3
  <Cmd_Switch> : Inport  Port=4
  Gain4 : Gain  Gain=1.7339
  Saturation1 : Saturate  UpperLimit=30*(pi/180)  LowerLimit=-30*(pi/180)
  Switch1 : Switch  Criteria=u2 > Threshold  Threshold=.5
  delta psi (shortest angle to chi) : MATLAB Function  TreatAsAtomicUnit=on
  Phi_cmd : Outport
  wires:
  chi_cmd/1 -> delta psi (shortest angle to chi)/1(chi_cmd)
  delta psi (shortest angle to chi)/1(d_chi) -> Gain4/1
  Gain4/1 -> Saturation1/1
  chi/1 -> delta psi (shortest angle to chi)/2(chi)
  Saturation1/1 -> Switch1/1
  Switch1/1 -> Phi_cmd/1
  <Cmd_Switch>/1 -> Switch1/2
  xi_pilot/1 -> Switch1/3

== system controllermodel/FCS/Controller/Heading controller/Lateral Base Controller ==
  Phi_e : Inport
  xi_pilot : Inport  Port=2
  <Cmd_Switch> : Inport  Port=3
  Gain6 : Gain  Gain=-0.0369
  Saturation5 : Saturate  UpperLimit=45*(pi/180)  LowerLimit=-45*(pi/180)
  Switch1 : Switch  Criteria=u2 > Threshold  Threshold=.5
  xi_cmd : Outport
  wires:
  Phi_e/1 -> Gain6/1
  Gain6/1 -> Saturation5/1  "xi_cmd"
  <Cmd_Switch>/1 -> Switch1/2
  Switch1/1 -> xi_cmd/1
  xi_pilot/1 -> Switch1/3
  Saturation5/1 -> Switch1/1

== system controllermodel/FCS/Controller/Heading controller/Roll damper ==
  xi : Inport
  p_IMU : Inport  Port=2
  Controller_Switch : Inport  Port=3
  Gain : Gain  Gain=-0.0027
  Sum : Sum  Inputs=|+-
  Switch1 : Switch  Criteria=u2 > Threshold  Threshold=.5
  xi_cmd : Outport
  wires:
  p_IMU/1 -> Gain/1
  Gain/1 -> Sum/2
  Sum/1 -> Switch1/1
  xi/1 -> Switch1/3, Sum/1
  Switch1/1 -> xi_cmd/1
  Controller_Switch/1 -> Switch1/2

== system controllermodel/FCS/Controller/Velocity controller/Velocity controller ==
  V_e : Inport
  thrust_pilot : Inport  Port=2
  <Cmd_Switch> : Inport  Port=3
  PID Controller2 : pid_lib/PID Controller  Controller=PI  Form=Parallel  TimeDomain=Discrete-time  UseExternalTs=off  SampleTime=0.01  IntegratorMethod=Forward Euler  FilterMethod=Forward Euler  ControllerParametersSource=internal  P=0.4443  I=0.6142  D=0  UseFilter=on  N=100  TunerSelectOption=Transfer Function Based (PID Tuner App)  InitialConditionSource=internal  InitialConditionForIntegrator=0.906230450117421  InitialConditionForFilter=0  DifferentiatorICPrevScaledInput=0  ExternalReset=none  TrackingMode=off  Kt=1  LimitOutput=on  SatLimitsSource=internal  UpperSaturationLimit=1  LowerSaturationLimit=0  LinearizeAsGain=on  AntiWindupMode=back-calculation  Kb=1  POutMin=[]  POutMax=[]  IOutMin=[]  IOutMax=[]  DOutMin=[]  DOutMax=[]  NOutMin=[]  NOutMax=[]  SumOutMin=[]  SumOutMax=[]  SaturationOutMin=[]  SaturationOutMax=[]  PParamMin=[]  PParamMax=[]  IParamMin=[]  IParamMax=[]  DParamMin=[]  DParamMax=[]  NParamMin=[]  NParamMax=[]  KbParamMin=[]  KbParamMax=[]  KtParamMin=[]  KtParamMax=[]  KbOutMin=[]  KbOutMax=[]  KtOutMin=[]  KtOutMax=[]  IntegratorOutMin=[]  IntegratorOutMax=[]  FilterOutMin=[]  FilterOutMax=[]  SumI1OutMin=[]  SumI1OutMax=[]  SumI2OutMin=[]  SumI2OutMax=[]  SumI3OutMin=[]  SumI3OutMax=[]  SumI4OutMin=[]  SumI4OutMax=[]  SumDOutMin=[]  SumDOutMax=[]  DifferentiatorOutMin=[]  DifferentiatorOutMax=[]  FilterDiffOutCoefMin=[]  FilterDiffOutCoefMax=[]  ReciprocalOutMin=[]  ReciprocalOutMax=[]  SumDenOutMin=[]  SumDenOutMax=[]  SumNumOutMin=[]  SumNumOutMax=[]  DivideOutMin=[]  DivideOutMax=[]  UdiffTsProdOutMin=[]  UdiffTsProdOutMax=[]  NTsProdOutMin=[]  NTsProdOutMax=[]  UintegralTsProdOutMin=[]  UintegralTsProdOutMax=[]  UngainTsProdOutMin=[]  UngainTsProdOutMax=[]  IntegratorContinuousStateAttributes=''  IntegratorStateMustResolveToSignalObject=off  IntegratorRTWStateStorageClass=Auto  FilterContinuousStateAttributes=''  FilterStateMustResolveToSignalObject=off  FilterRTWStateStorageClass=Auto  ParallelPVariant=InternalParameters  IdealPVariant=Disabled  IVariant=InternalParameters  DVariant=Disabled  IntegratorVariant=Discrete  SatVariant=Enabled  AWVariant=BackCalculation  PCopyVariant=Disabled  TRVariant=Disabled  FdbkBlocksVariant=Forward  IdealPFdbkVariant=Disabled  SatFdbkVariant=Disabled  DerivativeFilterVariant=Disabled  NVariant=Disabled  NCopyVariant=Disabled_SignalSpec  FilterICVariant=Disabled  IntegratorICVariant=InternalICs  ExternalResetVariant=Disabled  TRSumVariant=Passthrough  SumFdbkVariant=Disabled  SumVariant=Sum_PI  TsampFilterVariant=InternalTs  TsampNgainVariant=Passthrough  TsampIntegralVariant=Passthrough  ExternalSaturationOutDataTypeStr=Inherit: Same as second input
  Switch1 : Switch  Criteria=u2 > Threshold  Threshold=.5
  Thrust : Outport
  wires:
  V_e/1 -> PID Controller2/1
  Switch1/1 -> Thrust/1
  <Cmd_Switch>/1 -> Switch1/2
  thrust_pilot/1 -> Switch1/3
  PID Controller2/1 -> Switch1/1

== matlab function controllermodel/FCS/Controller/Waypoint controller (Azimuth and Distance calculator)/Waypoint selector ==
  data: R input; WP_LAT output; WP_LON output; n input; n output; V_cmd output; H_cmd output
function [WP_LAT,WP_LON,n,V_cmd,H_cmd] = fcn(R,n)

WP_initial = [52.50395966 13.17136002];      
WP =   [52.505314 13.173436 17 60;
        52.506339 13.167899 15 50;
        52.504314 13.167917 16 75;
        52.506696 13.173369 17 100;
        52.507362 13.171169 17 60;
        52.503816 13.171263 17 60;
        52.505314 13.173436 17 60];     
 
%% Switch between Waypoints    
if R < 20
    n = n + 1;    
    if n > 7    
        n = n - 1;        
    else        
        n = n;        
    end    
else    
    n = n;    
end

WP_LAT  = WP(n,1);
WP_LON  = WP(n,2);
V_cmd   = WP(n,3);
H_cmd   = WP(n,4);

== matlab function controllermodel/FCS/Controller/Waypoint controller (Azimuth and Distance calculator)/atan2 ==
  data: dy input; chi output; dx input
function chi = fcn(dy, dx)

if dx > 0 
    
    chi = atan(dy/dx);
        
elseif dx < 0 && dy >= 0
        
    chi = atan(dy/dx) + pi;
         
elseif dx < 0 && dy < 0
        
    chi = atan(dy/dx) - pi;  
    
elseif dx == 0 && dy > 0
        
    chi = +pi/2;    
    
elseif dx == 0 && dy < 0
        
    chi = -pi/2;     
    
    else 
        
    chi = 0;   
    
end
        
chi = chi;

== matlab function controllermodel/FCS/Controller/Heading controller/Heading Controller/delta psi (shortest angle to chi) ==
  data: chi_cmd input; chi input; d_chi output
function d_chi = fcn(chi_cmd, chi)

d_chi = mod(chi_cmd - chi + pi,2*pi) - pi;
